simulink model "CP_ContrSys_NLin_a_n9464263_2019"  (R2019b)
settings: Solver=VariableStepAuto  StartTime=0.0  StopTime=10.0  RelTol=1e-3
values from neighbouring files (symbols this model uses):
  C = [1 0 0 0 ... (first row only)    [nonlinear_dynamics.m]
  K = place(A, B, [-3, -4, -5, -6])    [nonlinear_dynamics.m]
  x0 = [0.2 20*pi/180 0 0]'    [CP_ContrSys_a_MainFile_n9464263.m]    (also in CP_ContrSys_b_MainFile_n9464263.m = [0.2 200*pi/180 0 0]'; nonlinear_dynamics.m = [0 0 0 0]')
  x_bar = x_bar_a    [CP_ContrSys_a_MainFile_n9464263.m]    (also in CP_ContrSys_b_MainFile_n9464263.m = x_bar_b; nonlinear_dynamics.m = sym('x_bar_', [4, 1]))
settings Model: Creator=cal  LastModifiedBy=cal
settings DataIOCC: ExternalInput=[m M_c l g]  SaveFormat=Array

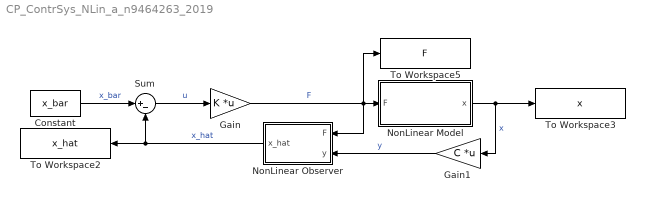
== system CP_ContrSys_NLin_a_n9464263_2019 ==
  Constant : Constant  Value=x_bar
  Gain : Gain  Gain=K  Multiplication=Matrix(K*u)
  Gain1 : Gain  Gain=C  Multiplication=Matrix(K*u)
  NonLinear Model : Subsystem
  NonLinear Observer : Subsystem
  Sum : Sum  Inputs=|+-
  To Workspace2 : ToWorkspace  VariableName=x_hat  SampleTime=-1
  To Workspace3 : ToWorkspace  VariableName=x  SampleTime=-1
  To Workspace5 : ToWorkspace  VariableName=F  SampleTime=-1
  wires:
  NonLinear Observer/1(x_hat) -> Sum/2, To Workspace2/1  "x_hat"
  Constant/1 -> Sum/1  "x_bar"
  NonLinear Model/1(x) -> To Workspace3/1, Gain1/1  "x"
  Gain1/1 -> NonLinear Observer/2(y)  "y"
  Sum/1 -> Gain/1  "u"
  Gain/1 -> NonLinear Observer/1(F), To Workspace5/1, NonLinear Model/1(F)  "F"

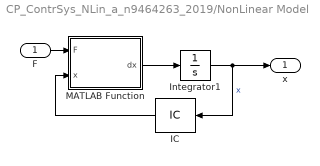
== system CP_ContrSys_NLin_a_n9464263_2019/NonLinear Model ==
  F : Inport
  IC : InitialCondition  Value=x0
  Integrator1 : Integrator
  MATLAB Function : MATLAB Function  TreatAsAtomicUnit=on
  x : Outport
  wires:
  IC/1 -> MATLAB Function/2(x)
  MATLAB Function/1(dx) -> Integrator1/1
  Integrator1/1 -> x/1, IC/1  "x"
  F/1 -> MATLAB Function/1(F)

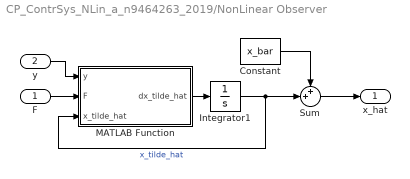
== system CP_ContrSys_NLin_a_n9464263_2019/NonLinear Observer ==
  F : Inport
  y : Inport  Port=2
  Constant : Constant  Value=x_bar
  Integrator1 : Integrator
  MATLAB Function : MATLAB Function  TreatAsAtomicUnit=on
  Sum : Sum  Inputs=++|
  x_hat : Outport
  wires:
  MATLAB Function/1(dx_tilde_hat) -> Integrator1/1
  Integrator1/1 -> MATLAB Function/3(x_tilde_hat), Sum/2  "x_tilde_hat"
  F/1 -> MATLAB Function/2(F)
  y/1 -> MATLAB Function/1(y)
  Constant/1 -> Sum/1
  Sum/1 -> x_hat/1

== matlab function CP_ContrSys_NLin_a_n9464263_2019/NonLinear Observer/MATLAB Function ==
  data: y input; F input; dx_tilde_hat output; x_tilde_hat input
function dx_tilde_hat = fcn(y, F, x_tilde_hat)
dx_tilde_hat = zeros(size(x_tilde_hat));
dx_tilde_hat = nonlinear_dynamics_observer(y, x_tilde_hat, F);

== matlab function CP_ContrSys_NLin_a_n9464263_2019/NonLinear Model/MATLAB Function ==
  data: F input; dx output; x input
function dx = fcn(F, x)
dx = zeros(size(x));
dx = nonlinear_dynamics_plant(x, F);
